simulink model "simulink224"  (R2020b)
settings: Solver=VariableStepAuto  StartTime=0.0  StopTime=1  RelTol=1e-3
libraries: dspsnks4 x1
settings Model: Creator=Nikita  LastModifiedBy=Nikita

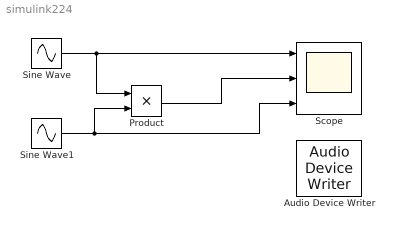
== system simulink224 ==
  Audio Device Writer : dspsnks4/Audio Device Writer  Driver=DirectSound  Device=Default  InheritSampleRate=on  SampleRate=44100  BitDepth=16-bit integer  BufferSize=4096  NumBuffers=10  DefaultOutputChannelMapping=on  OutputChannelMapping=1:2  OutputNumUnderrunSamples=off  DriverIdx=1  DeviceWarnFlag=''
  Product : Product
  Scope : Scope  NumInputPorts=3
  Sine Wave : Sin  SineType=Sample based  Frequency=2*pi*2  Samples=96  SampleTime=1/48000
  Sine Wave1 : Sin  SineType=Sample based  Frequency=2*pi*2  Samples=1536  SampleTime=1/48000
  wires:
  Sine Wave1/1 -> Scope/3, Product/2
  Product/1 -> Scope/2
  Sine Wave/1 -> Scope/1, Product/1
